simulink model "TA002"  (Simulink 6.3)
settings: Solver=ode45  StartTime=0.0  StopTime=0.5  RelTol=1e-3
undefined symbols (not defined in the file): a1, a2, a3, a4, a5, a6, a7, a8
libraries: powerlib_extras x2
settings Model: Creator=Phyo Mg Mg  LastModifiedBy=LT Phyo Mg Mg
settings OptimizationCC: InlineInvariantSignals=on

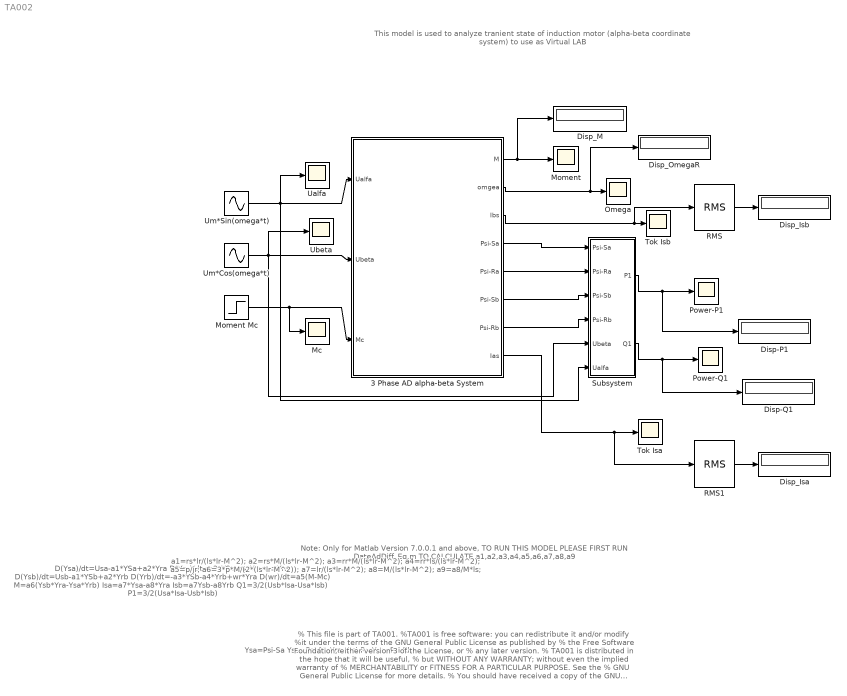
== system TA002 ==
  note: Note: Only for Matlab Version 7.0.0.1 and above,
      |
      | TO RUN THIS MODEL PLEASE FIRST RUN
      | DateAdDiff_Eq.m
      | TO CALCULATE a1,a2,a3,a4,a5,a6,a7,a8,a9
  note: D(Ysa)/dt=Usa-a1*YSa+a2*Yra
      | D(Yra)/dt=a3*YSa-a4*Yra-wr*Yra
      | D(Ysb)/dt=Usb-a1*YSb+a2*Yrb
      | D(Yrb)/dt=-a3*YSb-a4*Yrb+wr*Yra
      | D(wr)/dt=a5(M-Mc)
      | M=a6(Ysb*Yra-Ysa*Yrb)
      | Isa=a7*Ysa-a8*Yra
      | Isb=a7Ysb-a8Yrb
      | Q1=3/2(Usb*Isa-Usa*Isb)
      | P1=3/2(Usa*Isa-Usb*Isb)
  note: Ysa=Psi-Sa
      | Ysb=Psi-Sb
      | Yra=Psi-Ra
      | Yrb=Psi-Rb
  note: a1=rs*lr/(ls*lr-M^2);
      | a2=rs*M/(ls*lr-M^2);
      | a3=rr*M/(ls*lr-M^2);
      | a4=rr*ls/(ls*lr-M^2);
      | a5=p/jr;
      | a6=3*p*M/(2*(ls*lr-M^2));
      | a7=lr/(ls*lr-M^2);
      | a8=M/(ls*lr-M^2);
      | a9=a8/M*ls;
  note: % This file is part of TA001.
      | %TA001 is free software: you can redistribute it and/or modify
      | %it under the terms of the GNU General Public License as published by
      | % the Free Software Foundation, either version 3 of the License, or
      | % any later version.
      |
      | % TA001 is distributed in the hope that it will be useful,
      | % but WITHOUT ANY WARRANTY; without even the implied warranty of
      | % MERCHANTABILITY or FITNESS FOR A PARTICULAR PURPOSE.  See the
      | % GNU General Public License for more details.
      |
      | % You should have received a copy of the GNU General Public License
      | % along with TA001.  If not, see (http://www.gnu.org/licenses/).
  note: This model is used to analyze tranient state of induction motor (alpha-beta coordinate system)
      | to use as Virtual LAB
  3 Phase AD alpha-beta System : Subsystem
  Disp-P1 : Display
  Disp-Q1 : Display
  Disp_Isa : Display
  Disp_Isb : Display
  Disp_M : Display
  Disp_OmegaR : Display
  Mc : Scope
      settings: SaveName=ScopeData7
  Moment : Scope
  Moment Mc : Step  Time=0.08  After=17  SampleTime=0
  Omega : Scope
  Power-P1 : Scope
      settings: SaveName=ScopeData4
  Power-Q1 : Scope
      settings: SaveName=ScopeData3
  RMS : powerlib_extras/Measurements/RMS  f1=60
  RMS1 : powerlib_extras/Measurements/RMS  f1=60
  Subsystem : Subsystem
  Tok Isa : Scope
      settings: SaveName=ScopeData8
  Tok Isb : Scope
      settings: SaveName=ScopeData2
  Ualfa : Scope
      settings: SaveName=ScopeData5
  Ubeta : Scope
      settings: SaveName=ScopeData6
  "Um*Cos(omega*t) " : Sin  Amplitude=311.12  Frequency=314  Phase=pi/2  SampleTime=0
  Um*Sin(omega*t) : Sin  Amplitude=311.12  Frequency=314  SampleTime=0
  wires:
  Um*Sin(omega*t)/1 -> 3 Phase AD alpha-beta System/1(Ualfa), Subsystem/6(Ualfa), Ualfa/1
  "Um*Cos(omega*t) "/1 -> 3 Phase AD alpha-beta System/2(Ubeta), Subsystem/5(Ubeta), Ubeta/1
  Moment Mc/1 -> 3 Phase AD alpha-beta System/3(Mc), Mc/1
  3 Phase AD alpha-beta System/1(M) -> Moment/1, Disp_M/1
  3 Phase AD alpha-beta System/2(omgea) -> Omega/1, Disp_OmegaR/1
  3 Phase AD alpha-beta System/3(Ibs) -> Tok Isb/1, RMS/1
  RMS/1 -> Disp_Isb/1
  3 Phase AD alpha-beta System/4(Psi-Sa) -> Subsystem/1(Psi-Sa)
  3 Phase AD alpha-beta System/5(Psi-Ra) -> Subsystem/2(Psi-Ra)
  3 Phase AD alpha-beta System/6(Psi-Sb) -> Subsystem/3(Psi-Sb)
  3 Phase AD alpha-beta System/7(Psi-Rb) -> Subsystem/4(Psi-Rb)
  Subsystem/1(P1) -> Power-P1/1, Disp-P1/1
  Subsystem/2(Q1) -> Disp-Q1/1, Power-Q1/1
  RMS1/1 -> Disp_Isa/1
  3 Phase AD alpha-beta System/8(Ias) -> Tok Isa/1, RMS1/1

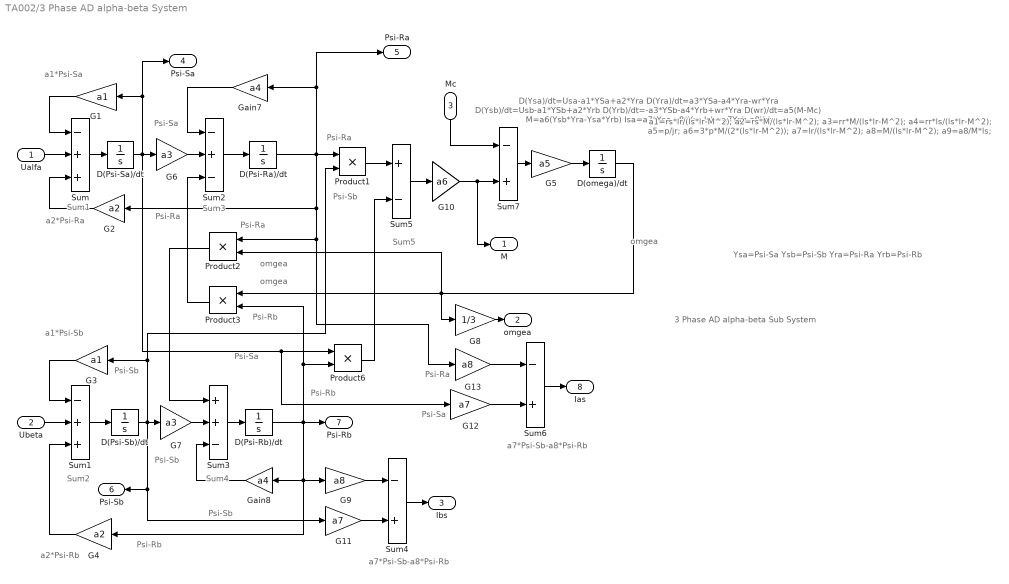
== system TA002/3 Phase AD alpha-beta System ==
  note: Sum3
  note: Sum4
  note: Sum5
  note: a7*Psi-Sb-a8*Psi-Rb
  note: Sum1
  note: Sum2
  note: Psi-Sa
  note: Psi-Sa
  note: Psi-Ra
  note: Psi-Ra
  note: omgea
  note: omgea
  note: omgea
  note: Psi-Rb
  note: Psi-Rb
  note: Psi-Rb
  note: Psi-Sb
  note: Psi-Sb
  note: Psi-Sb
  note: a1*Psi-Sa
  note: Psi-Ra
  note: a2*Psi-Ra
  note: a1*Psi-Sb
  note: a2*Psi-Rb
  note: Psi-Sb
  note: a7*Psi-Sb-a8*Psi-Rb
  note: Psi-Ra
  note: Psi-Sa
  note: D(Ysa)/dt=Usa-a1*YSa+a2*Yra
      | D(Yra)/dt=a3*YSa-a4*Yra-wr*Yra
      | D(Ysb)/dt=Usb-a1*YSb+a2*Yrb
      | D(Yrb)/dt=-a3*YSb-a4*Yrb+wr*Yra
      | D(wr)/dt=a5(M-Mc)
      | M=a6(Ysb*Yra-Ysa*Yrb)
      | Isa=a7*Ysa-a8*Yra
      | Isb=a7Ysb-a8Yrb
  note: Ysa=Psi-Sa
      | Ysb=Psi-Sb
      | Yra=Psi-Ra
      | Yrb=Psi-Rb
  note: a1=rs*lr/(ls*lr-M^2);
      | a2=rs*M/(ls*lr-M^2);
      | a3=rr*M/(ls*lr-M^2);
      | a4=rr*ls/(ls*lr-M^2);
      | a5=p/jr;
      | a6=3*p*M/(2*(ls*lr-M^2));
      | a7=lr/(ls*lr-M^2);
      | a8=M/(ls*lr-M^2);
      | a9=a8/M*ls;
  note: 3 Phase AD alpha-beta Sub System
  Ualfa : Inport
  Ubeta : Inport  Port=2
  Mc : Inport  Orientation=down  Port=3
  "D(Psi-Ra)/dt " : Integrator
  "D(Psi-Rb)/dt " : Integrator
  D(Psi-Sa)/dt : Integrator
  "D(Psi-Sb)/dt " : Integrator
  D(omega)/dt : Integrator
  G1 : Gain  Orientation=left  Gain=a1
  G10 : Gain  Gain=a6
  G11 : Gain  Gain=a7
  G12 : Gain  Gain=a7
  G13 : Gain  Gain=a8
  G2 : Gain  Orientation=left  Gain=a2
  G3 : Gain  Orientation=left  Gain=a1
  G4 : Gain  Orientation=left  Gain=a2
  G5 : Gain  Gain=a5
  G6 : Gain  Gain=a3
  G7 : Gain  Gain=a3
  G8 : Gain  Gain=1/3
  G9 : Gain  Gain=a8
  Gain7 : Gain  Orientation=left  Gain=a4
  Gain8 : Gain  Orientation=left  Gain=a4
  Product1 : Product  RndMeth=Zero
  Product2 : Product  Orientation=left  RndMeth=Zero
  Product3 : Product  Orientation=left  RndMeth=Zero
  Product6 : Product  RndMeth=Zero
  Sum : Sum  Inputs=-++
  Sum1 : Sum  Inputs=-++
  Sum2 : Sum  Inputs=-+-
  Sum3 : Sum  Inputs=++-
  Sum4 : Sum  Inputs=-+
  Sum5 : Sum  Inputs=+-
  Sum6 : Sum  Inputs=-+
  Sum7 : Sum  Inputs=-+
  M : Outport
  omgea : Outport  Port=2
  Ibs : Outport  Port=3
  Psi-Sa : Outport  Port=4
  Psi-Ra : Outport  Port=5
  Psi-Sb : Outport  Orientation=left  Port=6
  Psi-Rb : Outport  Port=7
  Ias : Outport  Port=8
  wires:
  Ualfa/1 -> Sum/2
  Ubeta/1 -> Sum1/2
  Mc/1 -> Sum7/1
  Sum/1 -> D(Psi-Sa)/dt/1
  G1/1 -> Sum/1
  G2/1 -> Sum/3
  G3/1 -> Sum1/1
  G4/1 -> Sum1/3
  D(Psi-Sa)/dt/1 -> G1/1, Psi-Sa/1, G6/1, Product6/1, G12/1
  "D(Psi-Sb)/dt "/1 -> G7/1, G3/1, Product1/2, G11/1, Psi-Sb/1
  Sum1/1 -> "D(Psi-Sb)/dt "/1
  G7/1 -> Sum3/2
  G6/1 -> Sum2/2
  Sum3/1 -> "D(Psi-Rb)/dt "/1
  Gain7/1 -> Sum2/1
  Sum2/1 -> "D(Psi-Ra)/dt "/1
  "D(Psi-Ra)/dt "/1 -> Product1/1, G2/1, Product2/1, G13/1, Gain7/1, Psi-Ra/1
  Product3/1 -> Sum2/3
  "D(Psi-Rb)/dt "/1 -> Psi-Rb/1, Gain8/1, G4/1, G9/1, Product6/2, Product3/2
  Gain8/1 -> Sum3/3
  G9/1 -> Sum4/1
  G11/1 -> Sum4/2
  Product1/1 -> Sum5/1
  Product6/1 -> Sum5/2
  Sum4/1 -> Ibs/1
  Sum5/1 -> G10/1
  G10/1 -> Sum7/2, M/1
  Sum7/1 -> G5/1
  G5/1 -> D(omega)/dt/1
  D(omega)/dt/1 -> Product2/2, Product3/1, G8/1
  G8/1 -> omgea/1
  Product2/1 -> Sum3/1
  G13/1 -> Sum6/1
  G12/1 -> Sum6/2
  Sum6/1 -> Ias/1

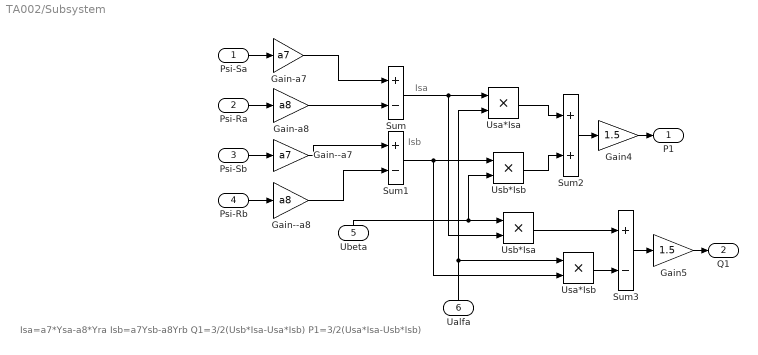
== system TA002/Subsystem ==
  note: Isa
  note: Isb
  note: Isa=a7*Ysa-a8*Yra
      | Isb=a7Ysb-a8Yrb
      | Q1=3/2(Usb*Isa-Usa*Isb)
      | P1=3/2(Usa*Isa-Usb*Isb)
  Psi-Sa : Inport
  Psi-Ra : Inport  Port=2
  Psi-Sb : Inport  Port=3
  Psi-Rb : Inport  Port=4
  Ubeta : Inport  Orientation=up  Port=5
  Ualfa : Inport  Orientation=up  Port=6
  Gain--a7 : Gain  Gain=a7
  Gain--a8 : Gain  Gain=a8
  Gain-a7 : Gain  Gain=a7
  Gain-a8 : Gain  Gain=a8
  Gain4 : Gain  Gain=1.5
  Gain5 : Gain  Gain=1.5
  Sum : Sum  Inputs=+-
  Sum1 : Sum  Inputs=+-
  Sum2 : Sum
  Sum3 : Sum  Inputs=+-
  Usa*Isa : Product  RndMeth=Zero
  Usa*Isb : Product  RndMeth=Zero
  Usb*Isa : Product  RndMeth=Zero
  Usb*Isb : Product  RndMeth=Zero
  P1 : Outport
  Q1 : Outport  Port=2
  wires:
  Gain-a7/1 -> Sum/1
  Gain-a8/1 -> Sum/2
  Gain--a7/1 -> Sum1/1
  Gain--a8/1 -> Sum1/2
  Sum/1 -> Usa*Isa/1, Usb*Isa/2
  Sum1/1 -> Usb*Isb/1, Usa*Isb/2
  Usa*Isa/1 -> Sum2/1
  Usb*Isb/1 -> Sum2/2
  Sum2/1 -> Gain4/1
  Sum3/1 -> Gain5/1
  Usb*Isa/1 -> Sum3/1
  Usa*Isb/1 -> Sum3/2
  Ubeta/1 -> Usb*Isb/2, Usb*Isa/1
  Ualfa/1 -> Usa*Isa/2, Usa*Isb/1
  Psi-Sa/1 -> Gain-a7/1
  Psi-Ra/1 -> Gain-a8/1
  Gain4/1 -> P1/1
  Psi-Sb/1 -> Gain--a7/1
  Psi-Rb/1 -> Gain--a8/1
  Gain5/1 -> Q1/1
